simulink model "FOSWEC_Heave"  (R2015b)
settings: Solver=ode4  StartTime=0  StopTime=10  FixedStep=0.05  RelTol=1e-3
undefined symbols (not defined in the file or in its folder): body, constraint
libraries: WECSim_Lib x21
settings Model: Creator=cmichel  LastModifiedBy=cmichel
settings DataIOCC: SaveFormat=Array
settings DebuggingCC: SolverPrmCheckMsg=warning
settings HardwareCC: ProdBitPerPointer=32  ProdLargestAtomicFloat=None  ProdIntDivRoundTo=Undefined  ProdEndianess=Unspecified  ProdWordSize=32  ProdHWDeviceType=32-bit Generic
settings GRTTargetCC: GeneratePreprocessorConditionals=Disable all
settings ConfigComp: CovModelRefEnable=Off  CovSFcnEnable=off

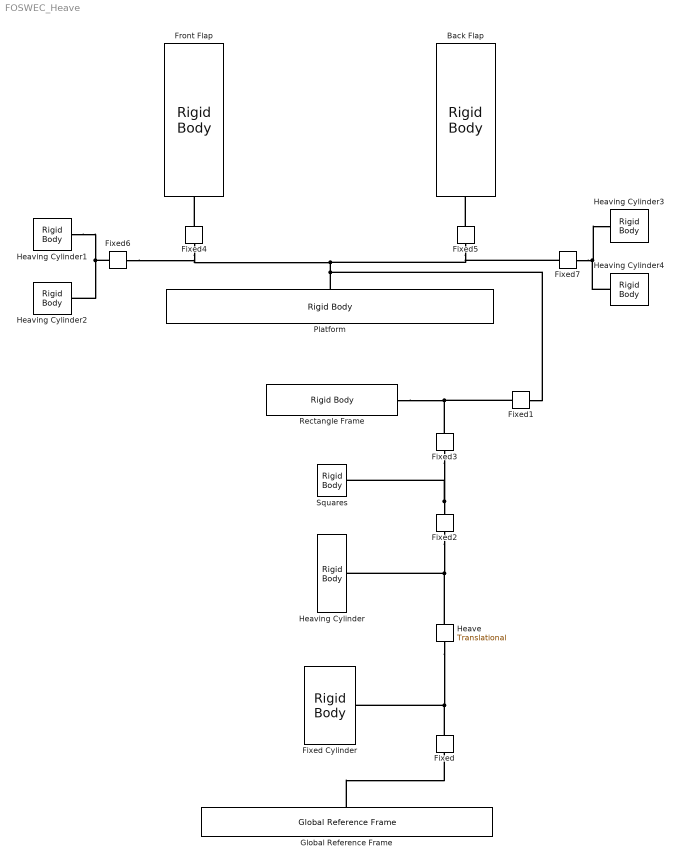
== system FOSWEC_Heave ==
  Back Flap : WECSim_Lib/Body Elements/Rigid Body  body=body(1)
      settings: AttributesFormatString=%<body>
  Fixed : WECSim_Lib/Constraints/Fixed  constraint=constraint(5)
      settings: AttributesFormatString=%<constraint>
  Fixed Cylinder : WECSim_Lib/Body Elements/Rigid Body  body=body(7)
      settings: AttributesFormatString=%<body>
  Fixed1 : WECSim_Lib/Constraints/Fixed  constraint=constraint(1)
      settings: AttributesFormatString=%<constraint>
  Fixed2 : WECSim_Lib/Constraints/Fixed  constraint=constraint(3)
      settings: AttributesFormatString=%<constraint>
  Fixed3 : WECSim_Lib/Constraints/Fixed  constraint=constraint(2)
      settings: AttributesFormatString=%<constraint>
  Fixed4 : WECSim_Lib/Constraints/Fixed  constraint=constraint(6)
      settings: AttributesFormatString=%<constraint>
  Fixed5 : WECSim_Lib/Constraints/Fixed  constraint=constraint(7)
      settings: AttributesFormatString=%<constraint>
  Fixed6 : WECSim_Lib/Constraints/Fixed  constraint=constraint(8)
      settings: AttributesFormatString=%<constraint>
  Fixed7 : WECSim_Lib/Constraints/Fixed  constraint=constraint(9)
      settings: AttributesFormatString=%<constraint>
  Front Flap : WECSim_Lib/Body Elements/Rigid Body  body=body(2)
      settings: AttributesFormatString=%<body>
  Global Reference Frame : WECSim_Lib/Frames/Global Reference Frame  waves=waves  simu=simu
  Heave : WECSim_Lib/Constraints/Translational  constraint=constraint(4)
      settings: AttributesFormatString=%<constraint>
  Heaving Cylinder : WECSim_Lib/Body Elements/Rigid Body  body=body(6)
      settings: AttributesFormatString=%<body>
  Heaving Cylinder1 : WECSim_Lib/Body Elements/Rigid Body  body=body(10)
      settings: AttributesFormatString=%<body>
  Heaving Cylinder2 : WECSim_Lib/Body Elements/Rigid Body  body=body(11)
      settings: AttributesFormatString=%<body>
  Heaving Cylinder3 : WECSim_Lib/Body Elements/Rigid Body  body=body(8)
      settings: AttributesFormatString=%<body>
  Heaving Cylinder4 : WECSim_Lib/Body Elements/Rigid Body  body=body(9)
      settings: AttributesFormatString=%<body>
  Platform : WECSim_Lib/Body Elements/Rigid Body  body=body(3)
      settings: AttributesFormatString=%<body>
  Rectangle Frame : WECSim_Lib/Body Elements/Rigid Body  body=body(4)
      settings: AttributesFormatString=%<body>
  Squares : WECSim_Lib/Body Elements/Rigid Body  body=body(5)
      settings: AttributesFormatString=%<body>
  connections:
  Fixed4/RConn1 -- Front Flap/RConn1
  Fixed5/RConn1 -- Back Flap/RConn1
  Platform/RConn1 -- Fixed1/RConn1 -- Fixed4/LConn1 -- Fixed6/LConn1 -- Fixed7/LConn1 -- Fixed5/LConn1
  Global Reference Frame/RConn1 -- Fixed/LConn1
  Fixed2/RConn1 -- Fixed3/LConn1 -- Squares/RConn1
  Fixed1/LConn1 -- Rectangle Frame/RConn1 -- Fixed3/RConn1
  Heave/RConn1 -- Heaving Cylinder/RConn1 -- Fixed2/LConn1
  Heave/LConn1 -- Fixed/RConn1 -- Fixed Cylinder/RConn1
  Heaving Cylinder1/RConn1 -- Fixed6/RConn1 -- Heaving Cylinder2/RConn1
  Heaving Cylinder4/RConn1 -- Fixed7/RConn1 -- Heaving Cylinder3/RConn1
